simulink model "Scope_Delay"  (R2020a)
settings: Solver=FixedStepAuto  StartTime=0.0  StopTime=inf  RelTol=1e-3  EnableMultiTasking=on
libraries: arduinolib x6, etargetslib x4
settings Model: SILPILModeSetting=veronly  ExtModeTrigDuration=2  Creator=imkis  LastModifiedBy=imkis
settings OptimizationCC: EnhancedBackFolding=on  PassReuseOutputArgsAs=Individual arguments  ZeroExternalMemoryAtStartup=off  ZeroInternalMemoryAtStartup=off  MaxStackSize=64  OptimizeBlockOrder=speed  DifferentSizesBufferReuse=on  OptimizationCustomize=off  EfficientTunableParamExpr=on
settings DebuggingCC: ParameterTunabilityLossMsg=error
settings HardwareCC: ProdBitPerInt=16  ProdBitPerPointer=16  ProdBitPerSizeT=16  ProdBitPerPtrDiffT=16  ProdLargestAtomicFloat=None  ProdWordSize=8  ProdHWDeviceType=Atmel->AVR
settings SFSimCC: MATLABDynamicMemAlloc=off
settings RTWCC: SystemTargetFile=ert.tlc  HardwareBoard=Arduino Mega 2560  TLCOptions=-aInlineSetEventsForThisBaseRateFcn=TLC_FALSE -aSuppressMultiTaskScheduler=TLC_FALSE -aRateBasedStepFcn=1  TemplateMakefile=ert_default_tmf  Toolchain=Arduino AVR  BuildConfiguration=Faster Runs
settings CodeAppCC: ForceParamTrailComments=on  IgnoreCustomStorageClasses=off  OperatorAnnotations=on  SimulinkDataObjDesc=on  SFDataObjDesc=on  InsertBlockDesc=on
settings ERTTargetCC: SupportContinuousTime=on  SupportVariableSizeSignals=on  ExtModeStaticAllocSize=2048

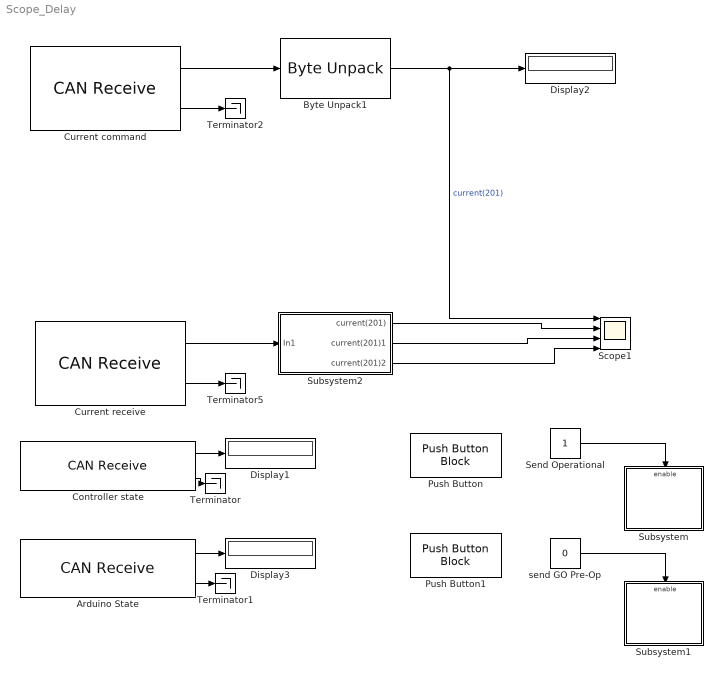
== system Scope_Delay ==
  Arduino State : arduinolib/CAN Receive  outputDataType=Raw data  identifierType=Standard (11-bit identifier)  messageId=hex2dec('702')  msgLength=1  SampleTime=1  outputError=off  outputRemote=off
      settings: SourceProductBaseCode=ARDUINO
  Byte Unpack1 : etargetslib/Byte Unpack  dimensions={[1]}  datatypes={'int16'}  byteAlign=2
  Controller state : arduinolib/CAN Receive  outputDataType=Raw data  identifierType=Standard (11-bit identifier)  messageId=hex2dec('701')  msgLength=1  SampleTime=1  outputError=off  outputRemote=off
      settings: SourceProductBaseCode=ARDUINO
  Current command : arduinolib/CAN Receive  outputDataType=Raw data  identifierType=Standard (11-bit identifier)  messageId=hex2dec('201')  msgLength=2  SampleTime=0.001  outputError=off  outputRemote=off
      settings: SourceProductBaseCode=ARDUINO
  Current receive : arduinolib/CAN Receive  outputDataType=Raw data  identifierType=Standard (11-bit identifier)  messageId=hex2dec('281')  msgLength=6  SampleTime=0.001  outputError=off  outputRemote=off
      settings: SourceProductBaseCode=ARDUINO
  Display1 : Display
  Display2 : Display
  Display3 : Display
  Push Button : PushButtonBlock  ButtonText=Go Operational
  Push Button1 : PushButtonBlock  ButtonText=GO Pre-Operational
  Scope1 : Scope  NumInputPorts=4
  Send Operational : Constant
  Subsystem : Subsystem
  Subsystem1 : Subsystem
  Subsystem2 : Subsystem
  Terminator{,1..2,5} (4 alike) : Terminator
  send GO Pre-Op : Constant  Value=0
  wires:
  Arduino State/2 -> Terminator1/1
  send GO Pre-Op/1 -> Subsystem1/Enable
  Controller state/1 -> Display1/1
  Send Operational/1 -> Subsystem/Enable
  Arduino State/1 -> Display3/1
  Controller state/2 -> Terminator/1
  Current command/2 -> Terminator2/1
  Byte Unpack1/1 -> Scope1/1, Display2/1  "current(201)"
  Current command/1 -> Byte Unpack1/1
  Subsystem2/3(current(201)2) -> Scope1/4
  Subsystem2/1(current(201)) -> Scope1/2
  Subsystem2/2(current(201)1) -> Scope1/3
  Current receive/2 -> Terminator5/1
  Current receive/1 -> Subsystem2/1(In1)

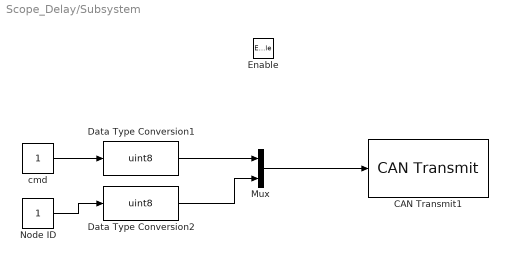
== system Scope_Delay/Subsystem ==
  Enable : EnablePort
  CAN Transmit1 : arduinolib/CAN Transmit  inputDataType=Raw data  BlockingMode_=off  BlockTimeout_=1  outputStatus=off  identifierType=Standard (11-bit identifier)  messageId=0  msgLength=2  remoteFrame=off
      settings: SourceProductBaseCode=ARDUINO
  Data Type Conversion1 : DataTypeConversion  OutDataTypeStr=uint8
  Data Type Conversion2 : DataTypeConversion  OutDataTypeStr=uint8
  Mux : Mux  Inputs=2
  Node ID : Constant  SampleTime=2
  cmd : Constant  SampleTime=2
  wires:
  Data Type Conversion2/1 -> Mux/2
  Data Type Conversion1/1 -> Mux/1
  Mux/1 -> CAN Transmit1/1
  Node ID/1 -> Data Type Conversion2/1
  cmd/1 -> Data Type Conversion1/1

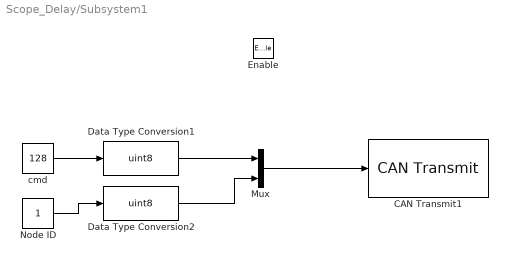
== system Scope_Delay/Subsystem1 ==
  Enable : EnablePort
  CAN Transmit1 : arduinolib/CAN Transmit  inputDataType=Raw data  BlockingMode_=off  BlockTimeout_=1  outputStatus=off  identifierType=Standard (11-bit identifier)  messageId=0  msgLength=2  remoteFrame=off
      settings: SourceProductBaseCode=ARDUINO
  Data Type Conversion1 : DataTypeConversion  OutDataTypeStr=uint8
  Data Type Conversion2 : DataTypeConversion  OutDataTypeStr=uint8
  Mux : Mux  Inputs=2
  Node ID : Constant  SampleTime=1
  cmd : Constant  Value=128  SampleTime=1
  wires:
  Data Type Conversion2/1 -> Mux/2
  Data Type Conversion1/1 -> Mux/1
  Mux/1 -> CAN Transmit1/1
  Node ID/1 -> Data Type Conversion2/1
  cmd/1 -> Data Type Conversion1/1

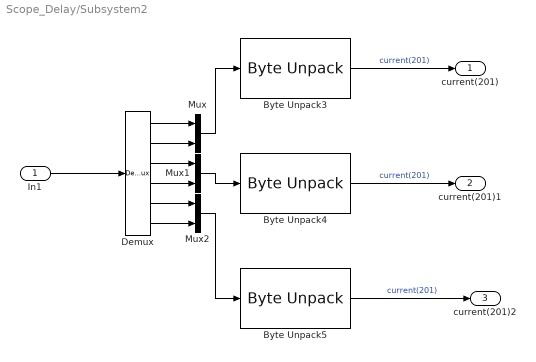
== system Scope_Delay/Subsystem2 ==
  In1 : Inport
  Byte Unpack3 : etargetslib/Byte Unpack  dimensions={[1]}  datatypes={'int16'}  byteAlign=2
  Byte Unpack4 : etargetslib/Byte Unpack  dimensions={[1]}  datatypes={'int16'}  byteAlign=2
  Byte Unpack5 : etargetslib/Byte Unpack  dimensions={[1]}  datatypes={'int16'}  byteAlign=2
  Demux : Demux  Outputs=6
  Mux : Mux  Inputs=2
  Mux1 : Mux  Inputs=2
  Mux2 : Mux  Inputs=2
  current(201) : Outport
  current(201)1 : Outport  Port=2
  current(201)2 : Outport  Port=3
  wires:
  Demux/6 -> Mux2/2
  Demux/5 -> Mux2/1
  Demux/1 -> Mux/1
  Mux/1 -> Byte Unpack3/1
  Demux/2 -> Mux/2
  Mux1/1 -> Byte Unpack4/1
  Demux/4 -> Mux1/2
  Mux2/1 -> Byte Unpack5/1
  Demux/3 -> Mux1/1
  Byte Unpack3/1 -> current(201)/1  "current(201)"
  Byte Unpack5/1 -> current(201)2/1  "current(201)"
  Byte Unpack4/1 -> current(201)1/1  "current(201)"
  In1/1 -> Demux/1
